simulink model "lablablab"  (R2019b)
settings: Solver=VariableStepAuto  StartTime=0.0  StopTime=100  RelTol=1e-3
settings Model: Creator=Abdurrahman  LastModifiedBy=Abdurrahman

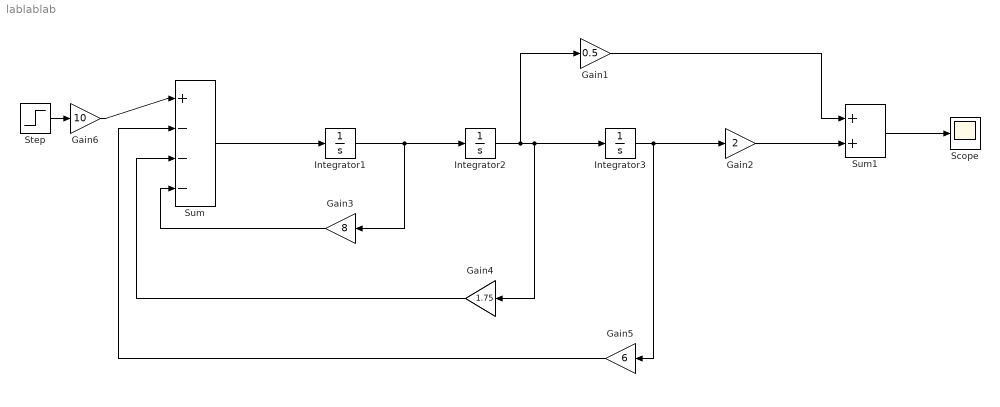
== system lablablab ==
  Gain1 : Gain  Gain=0.5
  Gain2 : Gain  Gain=2
  Gain3 : Gain  Gain=8
  Gain4 : Gain  Gain=1.75
  Gain5 : Gain  Gain=6
  Gain6 : Gain  Gain=10
  Integrator1 : Integrator
  Integrator2 : Integrator
  Integrator3 : Integrator
  Scope : Scope
  Step : Step  SampleTime=0
  Sum : Sum  Inputs=|+---
  Sum1 : Sum
  wires:
  Sum/1 -> Integrator1/1
  Integrator1/1 -> Gain3/1, Integrator2/1
  Integrator2/1 -> Gain1/1, Gain4/1, Integrator3/1
  Integrator3/1 -> Gain5/1, Gain2/1
  Step/1 -> Gain6/1
  Gain3/1 -> Sum/4
  Gain4/1 -> Sum/3
  Gain5/1 -> Sum/2
  Gain1/1 -> Sum1/1
  Gain2/1 -> Sum1/2
  Sum1/1 -> Scope/1
  Gain6/1 -> Sum/1
